simulink model "RALFMain"  (R2018b)
settings: Solver=FixedStepAuto  StartTime=0.0  StopTime=inf  RelTol=1e-3
InitFcn:
  | init
StopFcn:
  | stop
model workspace (MAT data in the model file):
  SL_ROS_VariableLengthArrays_MaxSizes.CommonInfo.ArrayTruncateAction = 'EmitWarning'
  SL_ROS_VariableLengthArrays_MaxSizes.MsgTypeMap = containers.Map
  SL_ROS_VariableLengthArrays_MaxSizes.MsgTypeMap.serialization.keys = {'sensor_msgs/Joy', 'std_msgs/Float32MultiArray', 'std_msgs/Int16MultiArray', 'std_msgs/Int32MultiArray', 'std_msgs/UInt16MultiArray', 'std_msgs/UInt8MultiArray'}
  SL_ROS_VariableLengthArrays_MaxSizes.MsgTypeMap.serialization.values{1}(1).PropertyName = 'Axes'
  SL_ROS_VariableLengthArrays_MaxSizes.MsgTypeMap.serialization.values{1}(1).DataType = 'single'
  SL_ROS_VariableLengthArrays_MaxSizes.MsgTypeMap.serialization.values{1}(1).MaxLength = 8
  SL_ROS_VariableLengthArrays_MaxSizes.MsgTypeMap.serialization.values{1}(2).PropertyName = 'Buttons'
  SL_ROS_VariableLengthArrays_MaxSizes.MsgTypeMap.serialization.values{1}(2).DataType = 'int32'
  SL_ROS_VariableLengthArrays_MaxSizes.MsgTypeMap.serialization.values{1}(2).MaxLength = 11
  SL_ROS_VariableLengthArrays_MaxSizes.MsgTypeMap.serialization.values{2}.PropertyName = 'Data'
  SL_ROS_VariableLengthArrays_MaxSizes.MsgTypeMap.serialization.values{2}.DataType = 'single'
  SL_ROS_VariableLengthArrays_MaxSizes.MsgTypeMap.serialization.values{2}.MaxLength = 8
  SL_ROS_VariableLengthArrays_MaxSizes.MsgTypeMap.serialization.values{3}.PropertyName = 'Data'
  SL_ROS_VariableLengthArrays_MaxSizes.MsgTypeMap.serialization.values{3}.DataType = 'int16'
  SL_ROS_VariableLengthArrays_MaxSizes.MsgTypeMap.serialization.values{3}.MaxLength = 4
  SL_ROS_VariableLengthArrays_MaxSizes.MsgTypeMap.serialization.values{4}.PropertyName = 'Data'
  SL_ROS_VariableLengthArrays_MaxSizes.MsgTypeMap.serialization.values{4}.DataType = 'int32'
  SL_ROS_VariableLengthArrays_MaxSizes.MsgTypeMap.serialization.values{4}.MaxLength = 8
  SL_ROS_VariableLengthArrays_MaxSizes.MsgTypeMap.serialization.values{5}.PropertyName = 'Data'
  SL_ROS_VariableLengthArrays_MaxSizes.MsgTypeMap.serialization.values{5}.DataType = 'uint16'
  SL_ROS_VariableLengthArrays_MaxSizes.MsgTypeMap.serialization.values{5}.MaxLength = 8
  SL_ROS_VariableLengthArrays_MaxSizes.MsgTypeMap.serialization.values{6}.PropertyName = 'Data'
  SL_ROS_VariableLengthArrays_MaxSizes.MsgTypeMap.serialization.values{6}.DataType = 'uint8'
  SL_ROS_VariableLengthArrays_MaxSizes.MsgTypeMap.serialization.values{6}.MaxLength = 8
  SL_ROS_VariableLengthArrays_MaxSizes.MsgTypeMap.serialization.uniformity = 0
  SL_ROS_VariableLengthArrays_MaxSizes.MsgTypeMap.serialization.keyType = 'char'
  SL_ROS_VariableLengthArrays_MaxSizes.MsgTypeMap.serialization.valueType = 'any'
values from neighbouring files (symbols this model uses):
  kp = 1    [init.m]
  nmax = 1500    [init.m]
  pwinkel = -1/20    (= -0.05)    [init.m]
  pwinkel_R = 0    [init.m]
libraries: simulink x9, etargetslib x5, cstblocks x4, simulink_extras x2, robotlib x2, realtime_pacer_lib x1
CloseFcn:
  | stop
settings Model: Creator=alf  LastModifiedBy=Systemtechnik Labor
settings DebuggingCC: ParameterPrecisionLossMsg=none

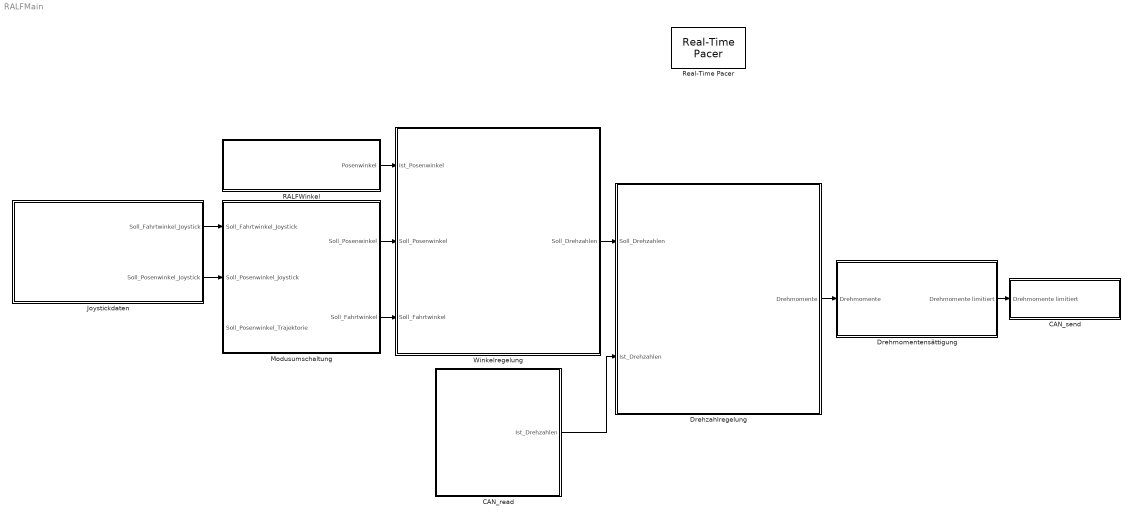
== system RALFMain ==
  CAN_read : Subsystem
  CAN_send : Subsystem
  Drehmomentensättigung : Subsystem
  Drehzahlregelung : Subsystem
  Joystickdaten : Subsystem
  Modusumschaltung : Subsystem
  RALFWinkel : Subsystem
  Real-Time Pacer : realtime_pacer_lib/Real-Time Pacer  simTimePerRealTime=1
  Winkelregelung : Subsystem
  wires:
  RALFWinkel/1(Posenwinkel) -> Winkelregelung/1(Ist_Posenwinkel)
  Modusumschaltung/1(Soll_Posenwinkel) -> Winkelregelung/2(Soll_Posenwinkel)
  Drehmomentensättigung/1(Drehmomente limitiert) -> CAN_send/1(Drehmomente limitiert)
  Modusumschaltung/2(Soll_Fahrtwinkel) -> Winkelregelung/3(Soll_Fahrtwinkel)
  Joystickdaten/1(Soll_Fahrtwinkel_Joystick) -> Modusumschaltung/1(Soll_Fahrtwinkel_Joystick)
  Joystickdaten/2(Soll_Posenwinkel_Joystick) -> Modusumschaltung/2(Soll_Posenwinkel_Joystick)
  Winkelregelung/1(Soll_Drehzahlen) -> Drehzahlregelung/1(Soll_Drehzahlen)
  CAN_read/1(Ist_Drehzahlen) -> Drehzahlregelung/2(Ist_Drehzahlen)
  Drehzahlregelung/1(Drehmomente) -> Drehmomentensättigung/1(Drehmomente)

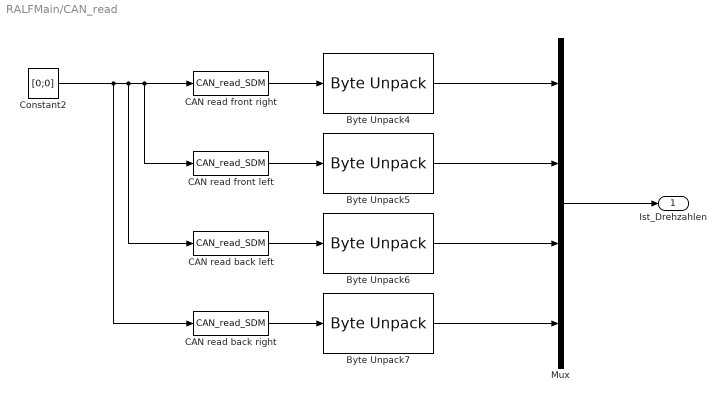
== system RALFMain/CAN_read ==
  Byte Unpack{4..7} (4 alike) : etargetslib/Byte Unpack  dimensions={[1]}  datatypes={'int16'}  byteAlign=1
  CAN read back left : S-Function  FunctionName=CAN_read_SDM  Parameters=Port,Identifier  SFunctionModules=socketcan  SFunctionDeploymentMode=off  EnableBusSupport=off  mask{Port=can0, Identifier=hex2dec('123')}
      mask prompts: Port "CAN Port"
      mask TypeOptions Port: can0 | can1 | can2
      mask DialogControl DescTextVar Prompt: Dennis Hotze, Dominik Eickmann
  CAN read back right : S-Function  FunctionName=CAN_read_SDM  Parameters=Port,Identifier  SFunctionModules=socketcan  SFunctionDeploymentMode=off  EnableBusSupport=off  mask{Port=can0, Identifier=hex2dec('133')}
      mask prompts: Port "CAN Port"
      mask TypeOptions Port: can0 | can1 | can2
      mask DialogControl DescTextVar Prompt: Dennis Hotze, Dominik Eickmann
  CAN read front left : S-Function  FunctionName=CAN_read_SDM  Parameters=Port,Identifier  SFunctionModules=socketcan  SFunctionDeploymentMode=off  EnableBusSupport=off  mask{Port=can0, Identifier=hex2dec('113')}
      mask prompts: Port "CAN Port"
      mask TypeOptions Port: can0 | can1 | can2
      mask DialogControl DescTextVar Prompt: Dennis Hotze, Dominik Eickmann
  "CAN read front right " : S-Function  FunctionName=CAN_read_SDM  Parameters=Port,Identifier  SFunctionModules=socketcan  SFunctionDeploymentMode=off  EnableBusSupport=off  mask{Port=can0, Identifier=hex2dec('103')}
      mask prompts: Port "CAN Port"
      mask TypeOptions Port: can0 | can1 | can2
      mask DialogControl DescTextVar Prompt: Dennis Hotze, Dominik Eickmann
  Constant2 : Constant  Value=[0;0]
  Mux : Mux
  Ist_Drehzahlen : Outport
  wires:
  "CAN read front right "/1 -> Byte Unpack4/1
  CAN read back left/1 -> Byte Unpack6/1
  CAN read front left/1 -> Byte Unpack5/1
  Constant2/1 -> CAN read back right/1, CAN read back left/1, CAN read front left/1, "CAN read front right "/1
  CAN read back right/1 -> Byte Unpack7/1
  Byte Unpack4/1 -> Mux/1
  Byte Unpack5/1 -> Mux/2
  Byte Unpack6/1 -> Mux/3
  Byte Unpack7/1 -> Mux/4
  Mux/1 -> Ist_Drehzahlen/1

== system RALFMain/CAN_send ==
  Drehmomente limitiert : Inport
  CAN send back left : S-Function  FunctionName=CAN_send  Parameters=Port,Identifier  SFunctionModules=socketcan  SFunctionDeploymentMode=off  EnableBusSupport=off  mask{Port=can0, Identifier=hex2dec('121')}
      mask prompts: Port "CAN Port"
      mask TypeOptions Port: can0 | can1 | can2
      mask DialogControl DescTextVar Prompt: Dennis Hotze, Dominik Eickmann
  CAN send back right : S-Function  FunctionName=CAN_send  Parameters=Port,Identifier  SFunctionModules=socketcan  SFunctionDeploymentMode=off  EnableBusSupport=off  mask{Port=can0, Identifier=hex2dec('131')}
      mask prompts: Port "CAN Port"
      mask TypeOptions Port: can0 | can1 | can2
      mask DialogControl DescTextVar Prompt: Dennis Hotze, Dominik Eickmann
  CAN send front left : S-Function  FunctionName=CAN_send  Parameters=Port,Identifier  SFunctionModules=socketcan  SFunctionDeploymentMode=off  EnableBusSupport=off  mask{Port=can0, Identifier=hex2dec('111')}
      mask prompts: Port "CAN Port"
      mask TypeOptions Port: can0 | can1 | can2
      mask DialogControl DescTextVar Prompt: Dennis Hotze, Dominik Eickmann
  CAN send front right : S-Function  FunctionName=CAN_send  Parameters=Port,Identifier  SFunctionModules=socketcan  SFunctionDeploymentMode=off  EnableBusSupport=off  mask{Port=can0, Identifier=hex2dec('101')}
      mask prompts: Port "CAN Port"
      mask TypeOptions Port: can0 | can1 | can2
      mask DialogControl DescTextVar Prompt: Dennis Hotze, Dominik Eickmann
  Demux : Demux
  wires:
  Demux/4 -> CAN send back right/1
  Demux/1 -> CAN send front right/1
  Demux/2 -> CAN send front left/1
  Demux/3 -> CAN send back left/1
  Drehmomente limitiert/1 -> Demux/1

== system RALFMain/Drehmomentensättigung ==
  Drehmomente : Inport
  Abfrage DMS-Betaetigung : Subsystem
  Byte Pack : etargetslib/Byte Pack  datatypes={'uint16'}  byteAlign=1
  Data Type Conversion : DataTypeConversion  OutDataTypeStr=uint16
  Product : Product
  Saturation : Saturate  UpperLimit=100  LowerLimit=-100
  Drehmomente limitiert : Outport
  wires:
  Byte Pack/1 -> Drehmomente limitiert/1
  Saturation/1 -> Data Type Conversion/1
  Data Type Conversion/1 -> Byte Pack/1
  Product/1 -> Saturation/1
  Drehmomente/1 -> Product/1
  Abfrage DMS-Betaetigung/1("DMS-Betaetigung ") -> Product/2

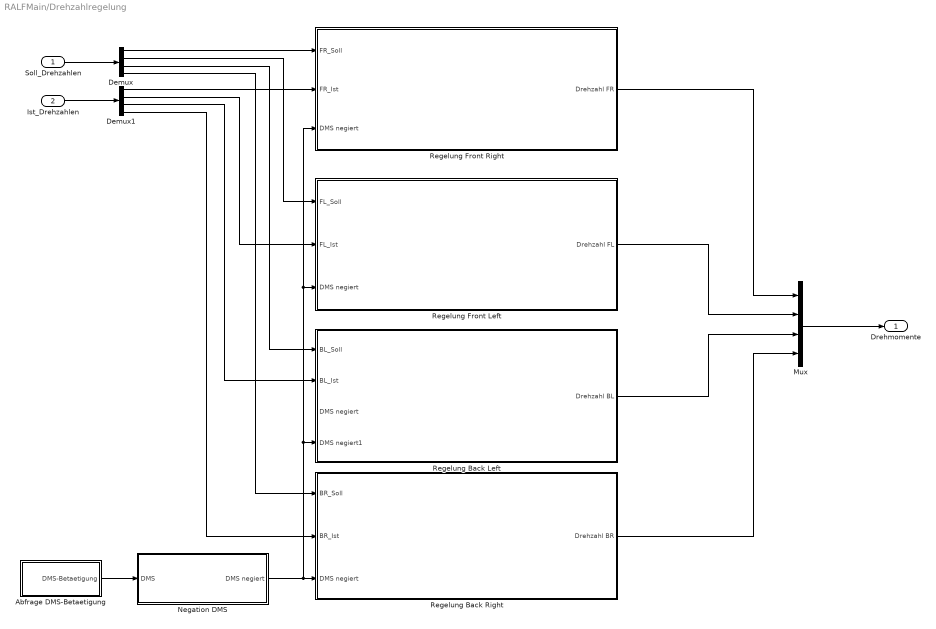
== system RALFMain/Drehzahlregelung ==
  Soll_Drehzahlen : Inport
  Ist_Drehzahlen : Inport  Port=2
  Abfrage DMS-Betaetigung : Subsystem
  Demux : Demux
  Demux1 : Demux
  Mux : Mux
  Negation DMS : Subsystem
  Regelung Back Left : Subsystem
  Regelung Back Right : Subsystem
  Regelung Front Left : Subsystem
  Regelung Front Right : Subsystem
  Drehmomente : Outport
  wires:
  Regelung Front Right/1(Drehzahl FR) -> Mux/1
  Demux/1 -> Regelung Front Right/1(FR_Soll)
  Demux1/1 -> Regelung Front Right/2(FR_Ist)
  Demux/2 -> Regelung Front Left/1(FL_Soll)
  Demux1/2 -> Regelung Front Left/2(FL_Ist)
  Regelung Front Left/1(Drehzahl FL) -> Mux/2
  Regelung Back Left/1(Drehzahl BL) -> Mux/3
  Demux1/3 -> Regelung Back Left/2(BL_Ist)
  Demux/3 -> Regelung Back Left/1(BL_Soll)
  Demux/4 -> Regelung Back Right/1(BR_Soll)
  Demux1/4 -> Regelung Back Right/2(BR_Ist)
  Negation DMS/1(DMS negiert) -> Regelung Back Right/3(DMS negiert), Regelung Front Left/3(DMS negiert), Regelung Front Right/3(DMS negiert), Regelung Back Left/4(DMS negiert1)
  Abfrage DMS-Betaetigung/1("DMS-Betaetigung ") -> Negation DMS/1(DMS)
  Soll_Drehzahlen/1 -> Demux/1
  Ist_Drehzahlen/1 -> Demux1/1
  Regelung Back Right/1(Drehzahl BR) -> Mux/4
  Mux/1 -> Drehmomente/1

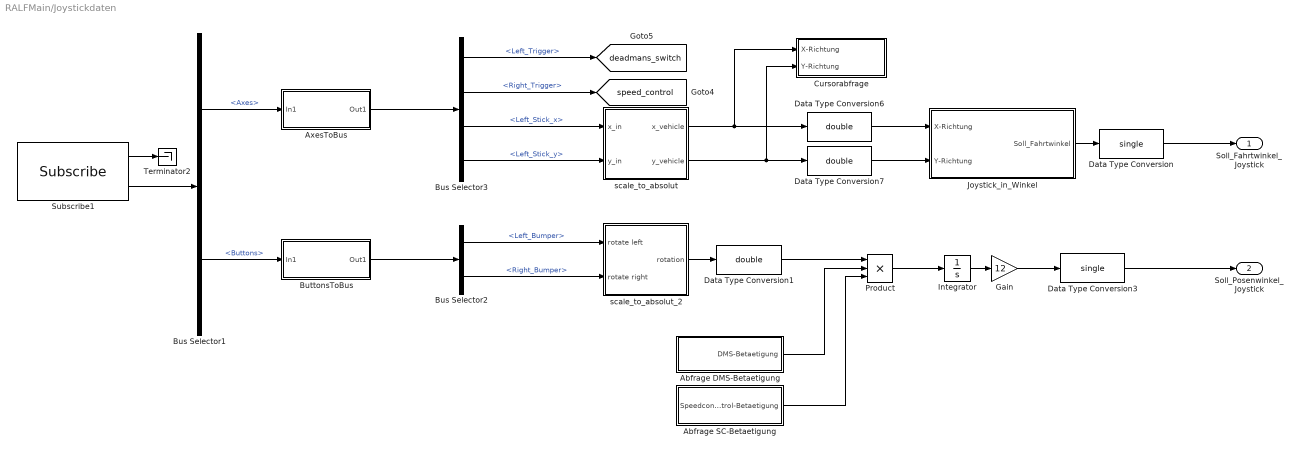
== system RALFMain/Joystickdaten ==
  Abfrage DMS-Betaetigung : Subsystem
  Abfrage SC-Betaetigung : Subsystem
  AxesToBus : Subsystem
  Bus Selector1 : BusSelector  OutputSignals=Axes,Buttons
  Bus Selector2 : BusSelector  OutputSignals=Bumper.Left_Bumper,Bumper.Right_Bumper
  Bus Selector3 : BusSelector  OutputSignals=Trigger.Left_Trigger,Trigger.Right_Trigger,Left_Stick.Left_Stick_x,Left_Stick.Left_Stick_y
  ButtonsToBus : Subsystem
  Cursorabfrage : Subsystem
  Data Type Conversion : DataTypeConversion  OutDataTypeStr=single
  Data Type Conversion1 : DataTypeConversion  OutDataTypeStr=double
  Data Type Conversion3 : DataTypeConversion  OutDataTypeStr=single
  Data Type Conversion6 : DataTypeConversion  OutDataTypeStr=double
  Data Type Conversion7 : DataTypeConversion  OutDataTypeStr=double
  Gain : Gain  Gain=12
  Integrator : Integrator
  Joystick_in_Winkel : Subsystem
  Product : Product  Inputs=3
  Subscribe1 : robotlib/Subscribe  topicSource=Select from ROS network  topic=/RALFJoy  messageType=sensor_msgs/Joy  sampleTime=-1  messageQueueLength=1
      settings: SourceProductBaseCode=RO
  Terminator2 : Terminator
  scale_to_absolut : Subsystem
  scale_to_absolut_2 : Subsystem
  Soll_Fahrtwinkel_Joystick : Outport
  Soll_Posenwinkel_Joystick : Outport  Port=2
  tag scope: deadmans_switch=global, speed_control=global
  wires:
  Bus Selector2/2 -> scale_to_absolut_2/2(rotate right)  "<Right_Bumper>"
  Bus Selector2/1 -> scale_to_absolut_2/1(rotate left)  "<Left_Bumper>"
  AxesToBus/1(Out1) -> Bus Selector3/1
  Bus Selector1/1 -> AxesToBus/1(In1)  "<Axes>"
  Bus Selector3/4 -> scale_to_absolut/2(y_in)  "<Left_Stick_y>"
  Subscribe1/2 -> Bus Selector1/1
  ButtonsToBus/1(Out1) -> Bus Selector2/1
  Bus Selector3/3 -> scale_to_absolut/1(x_in)  "<Left_Stick_x>"
  Bus Selector1/2 -> ButtonsToBus/1(In1)  "<Buttons>"
  Bus Selector3/2 -> [speed_control]  "<Right_Trigger>"
  Bus Selector3/1 -> [deadmans_switch]  "<Left_Trigger>"
  Subscribe1/1 -> Terminator2/1
  scale_to_absolut/1(x_vehicle) -> Cursorabfrage/1(X-Richtung), Data Type Conversion6/1
  Data Type Conversion7/1 -> Joystick_in_Winkel/2(Y-Richtung)
  Data Type Conversion6/1 -> Joystick_in_Winkel/1(X-Richtung)
  scale_to_absolut_2/1(rotation) -> Data Type Conversion1/1
  Data Type Conversion1/1 -> Product/1
  Product/1 -> Integrator/1
  Abfrage DMS-Betaetigung/1("DMS-Betaetigung ") -> Product/2
  Data Type Conversion/1 -> Soll_Fahrtwinkel_Joystick/1
  Joystick_in_Winkel/1(Soll_Fahrtwinkel) -> Data Type Conversion/1
  Data Type Conversion3/1 -> Soll_Posenwinkel_Joystick/1
  Integrator/1 -> Gain/1
  Gain/1 -> Data Type Conversion3/1
  Abfrage SC-Betaetigung/1("Speedcontrol-Betaetigung ") -> Product/3
  scale_to_absolut/2(y_vehicle) -> Cursorabfrage/2(Y-Richtung), Data Type Conversion7/1

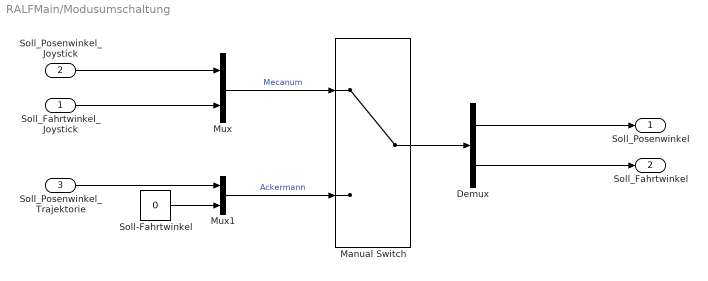
== system RALFMain/Modusumschaltung ==
  Soll_Fahrtwinkel_Joystick : Inport
  Soll_Posenwinkel_Joystick : Inport  Port=2
  Soll_Posenwinkel_Trajektorie : Inport  Port=3
  Demux : Demux  Outputs=2
  Manual Switch : ManualSwitch
  Mux : Mux  Inputs=2
  Mux1 : Mux  Inputs=2
  Soll-Fahrtwinkel : Constant  Value=0  OutDataTypeStr=single
  Soll_Posenwinkel : Outport
  Soll_Fahrtwinkel : Outport  Port=2
  wires:
  Manual Switch/1 -> Demux/1
  Demux/2 -> Soll_Fahrtwinkel/1
  Demux/1 -> Soll_Posenwinkel/1
  Soll-Fahrtwinkel/1 -> Mux1/2
  Soll_Posenwinkel_Joystick/1 -> Mux/1
  Soll_Posenwinkel_Trajektorie/1 -> Mux1/1
  Soll_Fahrtwinkel_Joystick/1 -> Mux/2
  Mux/1 -> Manual Switch/1  "Mecanum"
  Mux1/1 -> Manual Switch/2  "Ackermann"

== system RALFMain/RALFWinkel ==
  Bus Selector4 : BusSelector  OutputSignals=Z
  Data Type Conversion : DataTypeConversion  OutDataTypeStr=single
  Subscribe2 : robotlib/Subscribe  topicSource=Select from ROS network  topic=/ralfwinkel  messageType=geometry_msgs/Point  sampleTime=-1  messageQueueLength=1
      settings: SourceProductBaseCode=RO
  Terminator1 : Terminator
  Posenwinkel : Outport
  wires:
  Subscribe2/1 -> Terminator1/1
  Subscribe2/2 -> Bus Selector4/1
  Data Type Conversion/1 -> Posenwinkel/1
  Bus Selector4/1 -> Data Type Conversion/1  "<Z>"

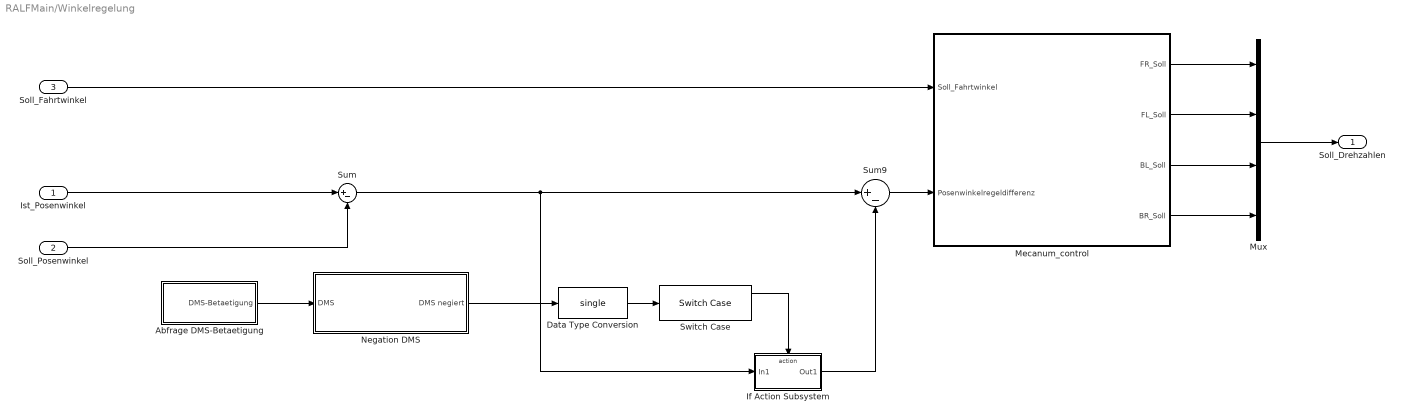
== system RALFMain/Winkelregelung ==
  Ist_Posenwinkel : Inport
  Soll_Posenwinkel : Inport  Port=2
  Soll_Fahrtwinkel : Inport  Port=3
  Abfrage DMS-Betaetigung : Subsystem
  Data Type Conversion : DataTypeConversion  OutDataTypeStr=single
  If Action Subsystem : Subsystem  TreatAsAtomicUnit=on
  Mecanum_control : Subsystem
  Mux : Mux
  Negation DMS : Subsystem
  Sum : Sum  Inputs=|+-
  Sum9 : Sum  Inputs=|+-
  Switch Case : SwitchCase
  Soll_Drehzahlen : Outport
  wires:
  Switch Case/1 -> If Action Subsystem/Action
  Data Type Conversion/1 -> Switch Case/1
  Soll_Posenwinkel/1 -> Sum/2
  If Action Subsystem/1(Out1) -> Sum9/2
  Soll_Fahrtwinkel/1 -> Mecanum_control/1(Soll_Fahrtwinkel)
  Sum9/1 -> Mecanum_control/2(Posenwinkelregeldifferenz)
  Negation DMS/1(DMS negiert) -> Data Type Conversion/1
  Abfrage DMS-Betaetigung/1("DMS-Betaetigung ") -> Negation DMS/1(DMS)
  Mecanum_control/1(FR_Soll) -> Mux/1
  Mecanum_control/4(BR_Soll) -> Mux/4
  Mecanum_control/2(FL_Soll) -> Mux/2
  Mecanum_control/3(BL_Soll) -> Mux/3
  Sum/1 -> If Action Subsystem/1(In1), Sum9/1
  Ist_Posenwinkel/1 -> Sum/1
  Mux/1 -> Soll_Drehzahlen/1

== system RALFMain/Drehmomentensättigung/Abfrage DMS-Betaetigung ==
  Compare To Constant : simulink/Logic and Bit Operations/Compare To Constant  relop=>  const=0.9  OutDataTypeStr=boolean
  Data Type Conversion : DataTypeConversion  OutDataTypeStr=single
  "DMS-Betaetigung " : Outport
  wires:
  Compare To Constant/1 -> Data Type Conversion/1
  Data Type Conversion/1 -> "DMS-Betaetigung "/1
  [deadmans_switch] -> Compare To Constant/1

== system RALFMain/Drehzahlregelung/Abfrage DMS-Betaetigung ==
  Compare To Constant : simulink/Logic and Bit Operations/Compare To Constant  relop=>  const=0.9  OutDataTypeStr=boolean
  Data Type Conversion : DataTypeConversion  OutDataTypeStr=single
  "DMS-Betaetigung " : Outport
  wires:
  Compare To Constant/1 -> Data Type Conversion/1
  Data Type Conversion/1 -> "DMS-Betaetigung "/1
  [deadmans_switch] -> Compare To Constant/1

== system RALFMain/Drehzahlregelung/Negation DMS ==
  DMS : Inport
  Constant : Constant  Value=-1
  Product1 : Product
  Sum4 : Sum  Inputs=|++
  DMS negiert : Outport
  wires:
  DMS/1 -> Sum4/1
  Constant/1 -> Product1/2, Sum4/2
  Sum4/1 -> Product1/1
  Product1/1 -> DMS negiert/1

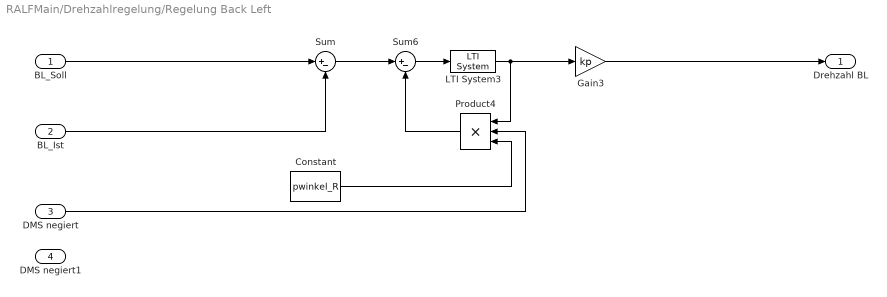
== system RALFMain/Drehzahlregelung/Regelung Back Left ==
  BL_Soll : Inport
  BL_Ist : Inport  Port=2
  DMS negiert : Inport  Port=3
  DMS negiert1 : Inport  Port=4
  Constant : Constant  Value=pwinkel_R
  Gain3 : Gain  Gain=kp
  LTI System3 : cstblocks/LTI System  sys=gpidv  IC=[]
  Product4 : Product  Inputs=3
  Sum : Sum  Inputs=|+-
  Sum6 : Sum  Inputs=|+-
  Drehzahl BL : Outport
  wires:
  Sum/1 -> Sum6/1
  Gain3/1 -> Drehzahl BL/1
  BL_Ist/1 -> Sum/2
  Constant/1 -> Product4/3
  DMS negiert/1 -> Product4/2
  Product4/1 -> Sum6/2
  Sum6/1 -> LTI System3/1
  BL_Soll/1 -> Sum/1
  LTI System3/1 -> Product4/1, Gain3/1

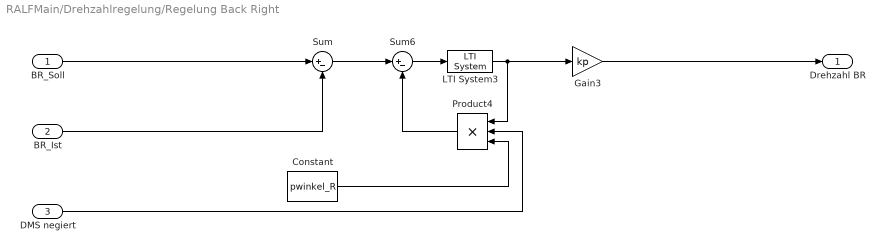
== system RALFMain/Drehzahlregelung/Regelung Back Right ==
  BR_Soll : Inport
  BR_Ist : Inport  Port=2
  DMS negiert : Inport  Port=3
  Constant : Constant  Value=pwinkel_R
  Gain3 : Gain  Gain=kp
  LTI System3 : cstblocks/LTI System  sys=gpidv  IC=[]
  Product4 : Product  Inputs=3
  Sum : Sum  Inputs=|+-
  Sum6 : Sum  Inputs=|+-
  Drehzahl BR : Outport
  wires:
  LTI System3/1 -> Product4/1, Gain3/1
  Sum/1 -> Sum6/1
  Gain3/1 -> Drehzahl BR/1
  Constant/1 -> Product4/3
  BR_Ist/1 -> Sum/2
  DMS negiert/1 -> Product4/2
  Sum6/1 -> LTI System3/1
  Product4/1 -> Sum6/2
  BR_Soll/1 -> Sum/1

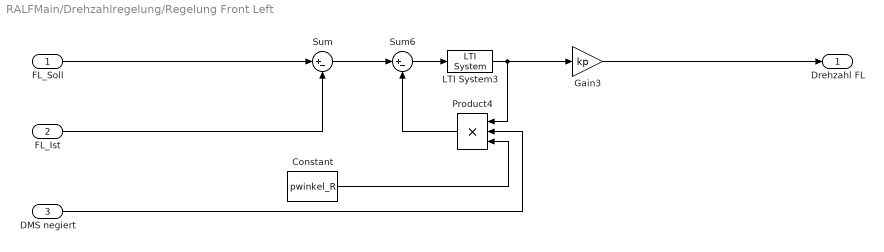
== system RALFMain/Drehzahlregelung/Regelung Front Left ==
  FL_Soll : Inport
  FL_Ist : Inport  Port=2
  DMS negiert : Inport  Port=3
  Constant : Constant  Value=pwinkel_R
  Gain3 : Gain  Gain=kp
  LTI System3 : cstblocks/LTI System  sys=gpidv  IC=[]
  Product4 : Product  Inputs=3
  Sum : Sum  Inputs=|+-
  Sum6 : Sum  Inputs=|+-
  Drehzahl FL : Outport
  wires:
  Sum/1 -> Sum6/1
  Gain3/1 -> Drehzahl FL/1
  FL_Ist/1 -> Sum/2
  Constant/1 -> Product4/3
  DMS negiert/1 -> Product4/2
  Product4/1 -> Sum6/2
  Sum6/1 -> LTI System3/1
  FL_Soll/1 -> Sum/1
  LTI System3/1 -> Product4/1, Gain3/1

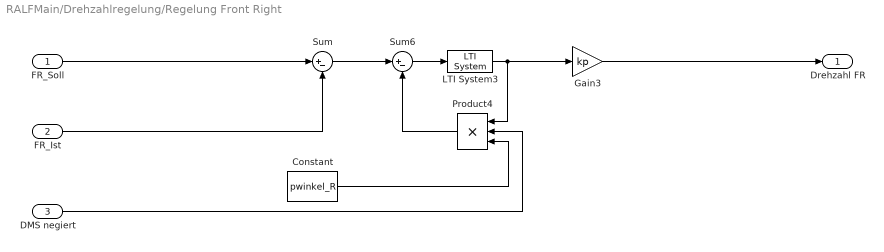
== system RALFMain/Drehzahlregelung/Regelung Front Right ==
  FR_Soll : Inport
  FR_Ist : Inport  Port=2
  DMS negiert : Inport  Port=3
  Constant : Constant  Value=pwinkel_R
  Gain3 : Gain  Gain=kp
  LTI System3 : cstblocks/LTI System  sys=gpidv  IC=[]
  Product4 : Product  Inputs=3
  Sum : Sum  Inputs=|+-
  Sum6 : Sum  Inputs=|+-
  Drehzahl FR : Outport
  wires:
  Gain3/1 -> Drehzahl FR/1
  LTI System3/1 -> Product4/1, Gain3/1
  Sum/1 -> Sum6/1
  FR_Ist/1 -> Sum/2
  Sum6/1 -> LTI System3/1
  FR_Soll/1 -> Sum/1
  Product4/1 -> Sum6/2
  Constant/1 -> Product4/3
  DMS negiert/1 -> Product4/2

== system RALFMain/Joystickdaten/Abfrage DMS-Betaetigung ==
  Compare To Constant : simulink/Logic and Bit Operations/Compare To Constant  relop=>  const=0.9  OutDataTypeStr=boolean
  Data Type Conversion : DataTypeConversion  OutDataTypeStr=single
  "DMS-Betaetigung " : Outport
  wires:
  Compare To Constant/1 -> Data Type Conversion/1
  Data Type Conversion/1 -> "DMS-Betaetigung "/1
  [deadmans_switch] -> Compare To Constant/1

== system RALFMain/Joystickdaten/Abfrage SC-Betaetigung ==
  Compare To Constant : simulink/Logic and Bit Operations/Compare To Constant  relop=>  const=0.9  OutDataTypeStr=boolean
  Data Type Conversion : DataTypeConversion  OutDataTypeStr=single
  "Speedcontrol-Betaetigung " : Outport
  wires:
  Compare To Constant/1 -> Data Type Conversion/1
  Data Type Conversion/1 -> "Speedcontrol-Betaetigung "/1
  [deadmans_switch] -> Compare To Constant/1

== system RALFMain/Joystickdaten/AxesToBus ==
  In1 : Inport
  Bus Creator{4..7} (4 alike) : BusCreator  Inputs=2
  Bus Creator8 : BusCreator  Inputs=4
  Demux : Demux  Outputs=8
  Out1 : Outport
  wires:
  Bus Creator4/1 -> Bus Creator8/1  "Left_Stick"
  Bus Creator5/1 -> Bus Creator8/3  "Right_Stick"
  Bus Creator6/1 -> Bus Creator8/2  "Trigger"
  Bus Creator7/1 -> Bus Creator8/4  "Direction_Pad"
  In1/1 -> Demux/1
  Demux/1 -> Bus Creator4/1  "Left_Stick_x"
  Demux/2 -> Bus Creator4/2  "Left_Stick_y"
  Demux/4 -> Bus Creator6/2  "Right_Trigger"
  Demux/3 -> Bus Creator6/1  "Left_Trigger"
  Demux/5 -> Bus Creator5/1  "Right_Stick_x"
  Demux/6 -> Bus Creator5/2  "Right_Stick_y"
  Demux/7 -> Bus Creator7/1  "Direction_Pad_x"
  Demux/8 -> Bus Creator7/2  "Direction_Pad_y"
  Bus Creator8/1 -> Out1/1

== system RALFMain/Joystickdaten/ButtonsToBus ==
  In1 : Inport
  Bus Creator : BusCreator  Inputs=6
  Bus Creator1 : BusCreator  Inputs=4
  Bus Creator2 : BusCreator  Inputs=2
  Bus Creator3 : BusCreator  Inputs=2
  Demux1 : Demux  Outputs=11
  Out1 : Outport
  wires:
  Demux1/9 -> Bus Creator/1  "XBOX_Guide_Button"
  Demux1/2 -> Bus Creator1/2  "B"
  Demux1/11 -> Bus Creator3/2  "Right_Stick"
  Demux1/10 -> Bus Creator3/1  "Left_Stick"
  Bus Creator3/1 -> Bus Creator/6  "Sticks"
  Bus Creator1/1 -> Bus Creator/4  "ABXY"
  Demux1/1 -> Bus Creator1/1  "A"
  Bus Creator2/1 -> Bus Creator/5  "Bumper"
  Demux1/7 -> Bus Creator/3  "Back_Button"
  Demux1/4 -> Bus Creator1/4  "Y"
  Demux1/3 -> Bus Creator1/3  "X"
  Demux1/6 -> Bus Creator2/2  "Right_Bumper"
  Demux1/8 -> Bus Creator/2  "Start_Button"
  Demux1/5 -> Bus Creator2/1  "Left_Bumper"
  In1/1 -> Demux1/1
  Bus Creator/1 -> Out1/1

== system RALFMain/Joystickdaten/Cursorabfrage ==
  X-Richtung : Inport
  Y-Richtung : Inport  Port=2
  Compare To Zero : simulink/Logic and Bit Operations/Compare To Zero  relop===  OutDataTypeStr=boolean
  Compare To Zero1 : simulink/Logic and Bit Operations/Compare To Zero  relop===  OutDataTypeStr=boolean
  Logical Operator : Logic  Operator=NAND  AllPortsSameDT=off  OutDataTypeStr=boolean
  tag scope: Cursor=global
  wires:
  X-Richtung/1 -> Compare To Zero/1
  Compare To Zero/1 -> Logical Operator/1
  Compare To Zero1/1 -> Logical Operator/2
  Logical Operator/1 -> [Cursor]
  Y-Richtung/1 -> Compare To Zero1/1

== system RALFMain/Joystickdaten/Joystick_in_Winkel ==
  X-Richtung : Inport
  Y-Richtung : Inport  Port=2
  Cartesian to Polar : simulink_extras/Transformations/Cartesian to Polar
      settings: SourceProductName=Simulink
  Soll_Fahrtwinkel : Outport
  wires:
  Cartesian to Polar/2 -> Soll_Fahrtwinkel/1
  X-Richtung/1 -> Cartesian to Polar/1
  Y-Richtung/1 -> Cartesian to Polar/2

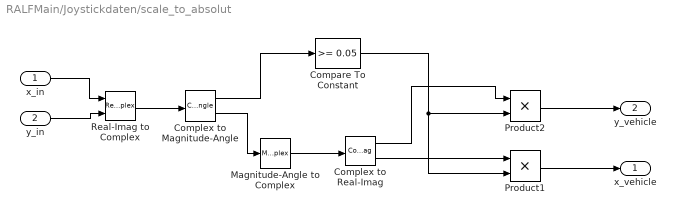
== system RALFMain/Joystickdaten/scale_to_absolut ==
  x_in : Inport
  y_in : Inport  Port=2
  Compare To Constant : simulink/Logic and Bit Operations/Compare To Constant  relop=>=  const=0.05  OutDataTypeStr=boolean
  Complex to Magnitude-Angle : ComplexToMagnitudeAngle
  Complex to Real-Imag : ComplexToRealImag
  Magnitude-Angle to Complex : MagnitudeAngleToComplex  Input=Angle  ConstantPart=1
  Product1 : Product
  Product2 : Product
  Real-Imag to Complex : RealImagToComplex
  x_vehicle : Outport
  y_vehicle : Outport  Port=2
  wires:
  Magnitude-Angle to Complex/1 -> Complex to Real-Imag/1
  Complex to Magnitude-Angle/2 -> Magnitude-Angle to Complex/1
  Product2/1 -> y_vehicle/1
  Compare To Constant/1 -> Product2/2, Product1/2
  Complex to Real-Imag/2 -> Product1/1
  Complex to Magnitude-Angle/1 -> Compare To Constant/1
  Real-Imag to Complex/1 -> Complex to Magnitude-Angle/1
  x_in/1 -> Real-Imag to Complex/1
  Complex to Real-Imag/1 -> Product2/1
  y_in/1 -> Real-Imag to Complex/2
  Product1/1 -> x_vehicle/1

== system RALFMain/Joystickdaten/scale_to_absolut_2 ==
  rotate left : Inport
  rotate right : Inport  Port=2
  Add : Sum
  Gain : Gain  Gain=-1  OutDataTypeStr=single
  rotation : Outport
  wires:
  rotate left/1 -> Gain/1
  Gain/1 -> Add/1
  rotate right/1 -> Add/2
  Add/1 -> rotation/1

== system RALFMain/Winkelregelung/Abfrage DMS-Betaetigung ==
  Compare To Constant : simulink/Logic and Bit Operations/Compare To Constant  relop=>  const=0.9  OutDataTypeStr=boolean
  Data Type Conversion : DataTypeConversion  OutDataTypeStr=single
  "DMS-Betaetigung " : Outport
  wires:
  Compare To Constant/1 -> Data Type Conversion/1
  Data Type Conversion/1 -> "DMS-Betaetigung "/1
  [deadmans_switch] -> Compare To Constant/1

== system RALFMain/Winkelregelung/If Action Subsystem ==
  In1 : Inport
  Action Port : ActionPort  ActionType=case
  Out1 : Outport
  wires:
  In1/1 -> Out1/1

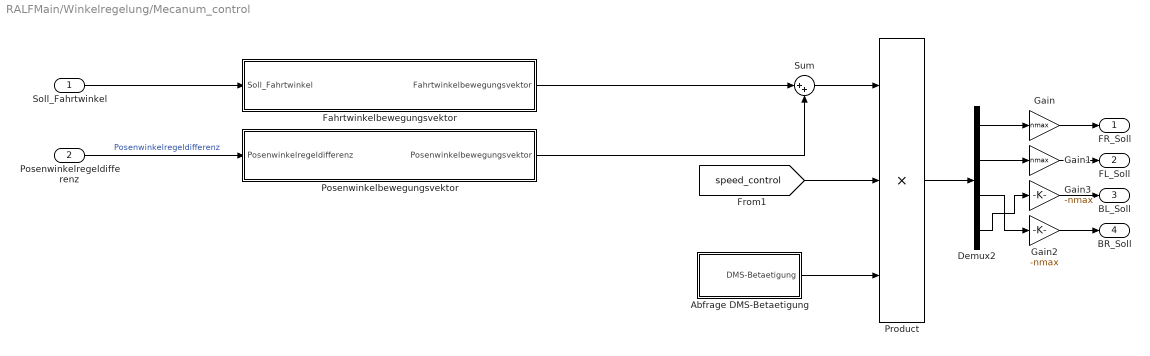
== system RALFMain/Winkelregelung/Mecanum_control ==
  Soll_Fahrtwinkel : Inport  OutDataTypeStr=single
  Posenwinkelregeldifferenz : Inport  Port=2  OutDataTypeStr=single
  Abfrage DMS-Betaetigung : Subsystem
  Demux2 : Demux
  Fahrtwinkelbewegungsvektor : Subsystem
  Gain : Gain  Gain=nmax  OutDataTypeStr=double
  Gain1 : Gain  Gain=nmax  OutDataTypeStr=double
  Gain2 : Gain  Gain=-nmax  OutDataTypeStr=double
  Gain3 : Gain  Gain=-nmax  OutDataTypeStr=double
  Posenwinkelbewegungsvektor : Subsystem
  Product : Product  Inputs=3  OutDataTypeStr=single
  Sum : Sum  Inputs=|++
  FR_Soll : Outport
  FL_Soll : Outport  Port=2
  BL_Soll : Outport  Port=3
  BR_Soll : Outport  Port=4
  wires:
  Product/1 -> Demux2/1
  Demux2/2 -> Gain1/1
  Demux2/1 -> Gain/1
  Gain3/1 -> BL_Soll/1
  Gain2/1 -> BR_Soll/1
  Gain1/1 -> FL_Soll/1
  Gain/1 -> FR_Soll/1
  Demux2/3 -> Gain2/1
  Demux2/4 -> Gain3/1
  [speed_control] -> Product/2
  Fahrtwinkelbewegungsvektor/1(Fahrtwinkelbewegungsvektor) -> Sum/1
  Sum/1 -> Product/1
  Abfrage DMS-Betaetigung/1("DMS-Betaetigung ") -> Product/3
  Posenwinkelregeldifferenz/1 -> Posenwinkelbewegungsvektor/1(Posenwinkelregeldifferenz)  "Posenwinkelregeldifferenz"
  Posenwinkelbewegungsvektor/1("Posenwinkelbewegungsvektor ") -> Sum/2
  Soll_Fahrtwinkel/1 -> Fahrtwinkelbewegungsvektor/1(Soll_Fahrtwinkel)

== system RALFMain/Winkelregelung/Negation DMS ==
  DMS : Inport
  Constant : Constant  Value=-1
  Product1 : Product
  Sum4 : Sum  Inputs=|++
  DMS negiert : Outport
  wires:
  DMS/1 -> Sum4/1
  Constant/1 -> Product1/2, Sum4/2
  Sum4/1 -> Product1/1
  Product1/1 -> DMS negiert/1

== system RALFMain/Winkelregelung/Mecanum_control/Abfrage DMS-Betaetigung ==
  Compare To Constant : simulink/Logic and Bit Operations/Compare To Constant  relop=>  const=0.9  OutDataTypeStr=boolean
  Data Type Conversion : DataTypeConversion  OutDataTypeStr=single
  "DMS-Betaetigung " : Outport
  wires:
  Compare To Constant/1 -> Data Type Conversion/1
  Data Type Conversion/1 -> "DMS-Betaetigung "/1
  [deadmans_switch] -> Compare To Constant/1

== system RALFMain/Winkelregelung/Mecanum_control/Fahrtwinkelbewegungsvektor ==
  Soll_Fahrtwinkel : Inport
  Constant : Constant  Value=[1 -1;1 1;1 1;1 -1]  OutDataTypeStr=single
  Data Type Conversion1 : DataTypeConversion  OutDataTypeStr=single
  Mux1 : Mux  Inputs=2
  Polar to Cartesian : simulink_extras/Transformations/Polar to Cartesian
      settings: SourceProductName=Simulink  SourceProductBaseCode=SL
  Product1 : Product  Multiplication=Matrix(*)
  Saturation3 : Saturate  UpperLimit=1  LowerLimit=-1
  Fahrtwinkelbewegungsvektor : Outport
  wires:
  Soll_Fahrtwinkel/1 -> Polar to Cartesian/2
  Polar to Cartesian/2 -> Mux1/2
  Constant/1 -> Product1/1
  Product1/1 -> Saturation3/1
  [Cursor] -> Data Type Conversion1/1
  Data Type Conversion1/1 -> Polar to Cartesian/1
  Polar to Cartesian/1 -> Mux1/1
  Mux1/1 -> Product1/2
  Saturation3/1 -> Fahrtwinkelbewegungsvektor/1

== system RALFMain/Winkelregelung/Mecanum_control/Posenwinkelbewegungsvektor ==
  Posenwinkelregeldifferenz : Inport
  Constant1 : Constant  Value=[-1;1;-1;1]  OutDataTypeStr=single
  Gain4 : Gain  Gain=pwinkel
  Product2 : Product  Multiplication=Matrix(*)
  "Posenwinkelbewegungsvektor " : Outport
  wires:
  Constant1/1 -> Product2/1
  Gain4/1 -> Product2/2
  Product2/1 -> "Posenwinkelbewegungsvektor "/1
  Posenwinkelregeldifferenz/1 -> Gain4/1
